simulink model "Model_2017_04_18"  (R2016a)
settings: Solver=VariableStepAuto  StartTime=0.0  StopTime=2  RelTol=1e-3
InitFcn:
  | parametriAM
values from neighbouring files (symbols this model uses):
  Imrn = 7.4    [parametriAM.m]
  Ismax = In*sqrt(2)    [parametriAM.m]
  J = 0.019    [parametriAM.m]    (also in podatki.m = 0.01)
  Ki_Imr = 1000    [parametriAM.m]
  Ki_tok = 5.0    (= 5)    [parametriAM.m]
  Kp_Imr = 100    [parametriAM.m]
  Kp_tok = 0.05    [parametriAM.m]
  Kp_wr = 50    [parametriAM.m]
  Lm = 0.0493    [parametriAM.m]    (also in podatki.m = 0.2342)
  Lr = 0.05315    [parametriAM.m]    (also in podatki.m = 0.2449)
  Ls = 0.05315    [parametriAM.m]    (also in podatki.m = 0.2449)
  Lst = sigma*Ls    (= 0.00742111947319)    [parametriAM.m]
  pp = 3    [parametriAM.m]    (also in podatki.m = 2)
  Rs = 0.594    [parametriAM.m]    (also in podatki.m = 3.7)
  sigma = 1 - 1/((1+sigmaR)*(1+sigmaS))    (= 0.13962595434)    [parametriAM.m]
  Tr = Lr/Rr    (= 0.0771407837446)    [parametriAM.m]
  Udc = Un*sqrt(2/3*2)    [parametriAM.m]
  wb_upper_limit_field_weaking = sqrt((Ls^2+Lst^2)/(2*Lst^2*Ls^2))*Un/Ismax    [parametriAM.m]
  wn = Udc/sqrt(Ls^2*(Imrn)^2+Lst^2*(Ismax^2-(Imrn)^2))    [maximalnaelipsa.m]    (also in parametriAM.m = Udc/sqrt(Ls^2*(Imrn)^2+Lst^2*(Ismax^2-(Imrn)^2))/pp/sqrt(2))
libraries: simulink x6
settings Model: Creator=Mitja1  LastModifiedBy=Mitja1

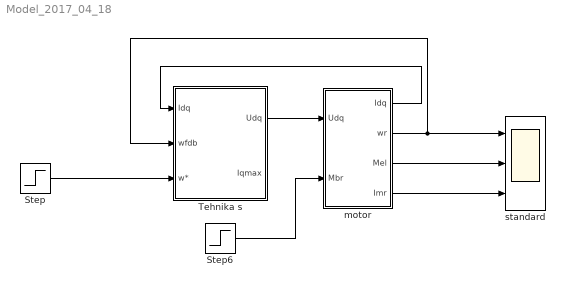
== system Model_2017_04_18 ==
  Step : Step  Time=0.05  After=4000/60*2*pi  SampleTime=0
  Step6 : Step  Time=0.5  After=2  SampleTime=0
  Tehnika s : Subsystem
  motor : Subsystem
  standard : Scope  NumInputPorts=3
  wires:
  motor/1(Idq) -> Tehnika s/1(Idq)
  motor/2(wr) -> Tehnika s/2(wfdb), standard/1
  motor/4(Imr) -> standard/3
  Tehnika s/1(Udq) -> motor/1(Udq)
  motor/3(Mel) -> standard/2
  Step6/1 -> motor/2(Mbr)
  Step/1 -> Tehnika s/3(w*)

== system Model_2017_04_18/Tehnika s ==
  Idq : Inport
  wfdb : Inport  Port=2
  w* : Inport  Port=3
  Gain2 : Gain  Gain=Udc
  M9 : ToWorkspace  VariableName=I_mr_sref  SampleTime=-1
      settings: Decimation=3  Save2DSignal=2-D array (concatenate along first dimension)
  Magnetilnireg : Subsystem
  Manual Switch : ManualSwitch
  Regulacija navora : Subsystem
  Subsystem : Subsystem
  Tok regulator : Subsystem
  Udq : Outport
  Iqmax : Outport  Port=2
  wires:
  Regulacija navora/1(iq*) -> Tok regulator/3(Iq)
  Regulacija navora/2(Iqmax) -> Iqmax/1
  Idq/1 -> Tok regulator/1(Idqdej), Regulacija navora/2(Idqdej), Subsystem/2(Idq), Magnetilnireg/1(Idqdej)
  w*/1 -> Subsystem/1(In1), Regulacija navora/1(w*)
  Tok regulator/1(Udq*) -> Gain2/1
  Gain2/1 -> Udq/1
  Magnetilnireg/1(Id*) -> Tok regulator/2(Id)
  Manual Switch/1 -> Magnetilnireg/2(Imr*)
  Subsystem/2(A) -> Manual Switch/1
  Subsystem/3(B) -> Manual Switch/2
  wfdb/1 -> Regulacija navora/3(wfdb)

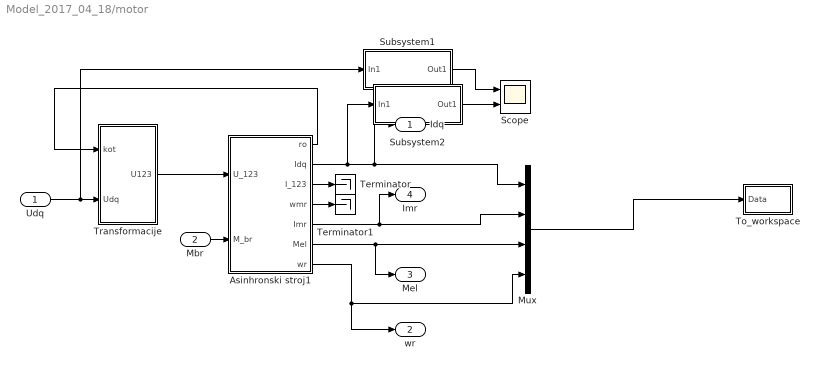
== system Model_2017_04_18/motor ==
  Udq : Inport
  Mbr : Inport  Port=2
  Asinhronski stroj1 : Subsystem  InitFcn=parametriAM
  Mux : Mux
  Scope : Scope  NumInputPorts=2
  Subsystem1 : Subsystem
  Subsystem2 : Subsystem
  Terminator : Terminator
  Terminator1 : Terminator
  To_workspace : Subsystem
  Transformacije : Subsystem
  Idq : Outport
  wr : Outport  Port=2
  Mel : Outport  Port=3
  Imr : Outport  Port=4
  wires:
  Mbr/1 -> Asinhronski stroj1/2(M_br)
  Asinhronski stroj1/6(Mel) -> Mux/3, Mel/1
  Asinhronski stroj1/7(wr) -> wr/1, Mux/4
  Asinhronski stroj1/5(Imr) -> Mux/2, Imr/1
  Udq/1 -> Subsystem1/1(In1), Transformacije/2(Udq)
  Transformacije/1(U123) -> Asinhronski stroj1/1(U_123)
  Asinhronski stroj1/1(ro) -> Transformacije/1(kot)
  Asinhronski stroj1/2(Idq) -> Subsystem2/1(In1), Idq/1, Mux/1
  Mux/1 -> To_workspace/1(Data)
  Asinhronski stroj1/4(wmr) -> Terminator1/1
  Asinhronski stroj1/3(I_123) -> Terminator/1
  Subsystem1/1(Out1) -> Scope/1
  Subsystem2/1(Out1) -> Scope/2

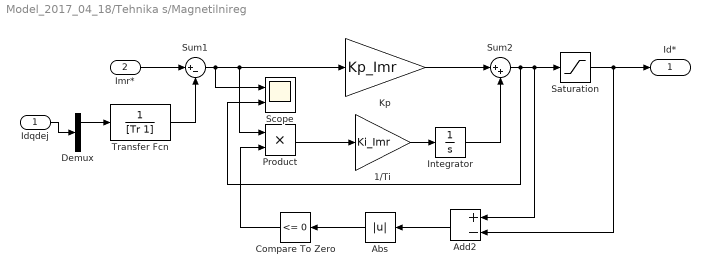
== system Model_2017_04_18/Tehnika s/Magnetilnireg ==
  Idqdej : Inport
  Imr* : Inport  Port=2
  1/Ti : Gain  Gain=Ki_Imr  SaturateOnIntegerOverflow=on  OutDataTypeStr=Inherit: Same as input  ParamDataTypeStr=Inherit: Same as input
  Abs : Abs  ZeroCross=off
  Add2 : Sum  Inputs=+-
  Compare To Zero : simulink/Logic and Bit Operations/Compare To Zero  relop=<=  OutDataTypeStr=boolean  ZeroCross=off
  Demux : Demux  Outputs=2
  Integrator : Integrator
  Kp : Gain  Gain=Kp_Imr  SaturateOnIntegerOverflow=on  OutDataTypeStr=Inherit: Same as input  ParamDataTypeStr=Inherit: Same as input
  Product : Product
  Saturation : Saturate  UpperLimit=Ismax  LowerLimit=-Ismax  ZeroCross=off
  Scope : Scope  NumInputPorts=2
  Sum1 : Sum  Inputs=|+-
  Sum2 : Sum  Inputs=|++
  Transfer Fcn : TransferFcn  Denominator=[Tr 1]
  Id* : Outport
  wires:
  Idqdej/1 -> Demux/1
  Transfer Fcn/1 -> Sum1/2
  Demux/1 -> Transfer Fcn/1
  Saturation/1 -> Id*/1, Add2/2
  Imr*/1 -> Sum1/1
  Integrator/1 -> Sum2/2
  Sum2/1 -> Saturation/1, Add2/1, Scope/2
  Compare To Zero/1 -> Product/2
  Kp/1 -> Sum2/1
  Product/1 -> 1/Ti/1
  1/Ti/1 -> Integrator/1
  Abs/1 -> Compare To Zero/1
  Add2/1 -> Abs/1
  Sum1/1 -> Kp/1, Product/1, Scope/1

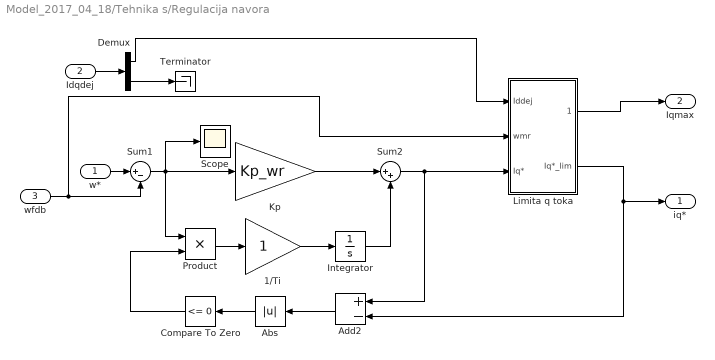
== system Model_2017_04_18/Tehnika s/Regulacija navora ==
  w* : Inport
  Idqdej : Inport  Port=2
  wfdb : Inport  Port=3
  1/Ti : Gain  SaturateOnIntegerOverflow=on  OutDataTypeStr=Inherit: Same as input  ParamDataTypeStr=Inherit: Same as input
  Abs : Abs
  Add2 : Sum  Inputs=+-
  Compare To Zero : simulink/Logic and Bit Operations/Compare To Zero  relop=<=  OutDataTypeStr=boolean
  Demux : Demux  Outputs=2
  Integrator : Integrator
  Kp : Gain  Gain=Kp_wr  SaturateOnIntegerOverflow=on  OutDataTypeStr=Inherit: Same as input  ParamDataTypeStr=Inherit: Same as input
  Limita q toka : Subsystem
  Product : Product
  Scope : Scope
  Sum1 : Sum  Inputs=|+-
  Sum2 : Sum  Inputs=|++
  Terminator : Terminator
  iq* : Outport
  Iqmax : Outport  Port=2
  wires:
  Demux/2 -> Terminator/1
  wfdb/1 -> Sum1/2, Limita q toka/2(wmr)
  Sum2/1 -> Add2/1, Limita q toka/3(Iq*)
  Demux/1 -> Limita q toka/1(Iddej)
  Limita q toka/1(Iqmaxlim) -> Iqmax/1
  Idqdej/1 -> Demux/1
  Limita q toka/2(Iq*_lim) -> Add2/2, iq*/1
  w*/1 -> Sum1/1
  Product/1 -> 1/Ti/1
  Compare To Zero/1 -> Product/2
  Kp/1 -> Sum2/1
  Abs/1 -> Compare To Zero/1
  Add2/1 -> Abs/1
  Integrator/1 -> Sum2/2
  Sum1/1 -> Scope/1, Kp/1, Product/1
  1/Ti/1 -> Integrator/1

== system Model_2017_04_18/Tehnika s/Subsystem ==
  In1 : Inport
  Idq : Inport  Port=2
  TechniqueA1 : Subsystem
  TechniqueA2 : Subsystem
  TechniqueB1 : Subsystem
  Nemec : Outport
  A : Outport  Port=2
  B : Outport  Port=3
  wires:
  In1/1 -> TechniqueA1/1(wmr), TechniqueB1/2(w), TechniqueA2/1(wmr)
  TechniqueA2/1(Nemec) -> Nemec/1
  Idq/1 -> TechniqueB1/1(Isdq)
  TechniqueB1/1(6.1-135) -> B/1
  TechniqueA1/1(6.1-126) -> A/1

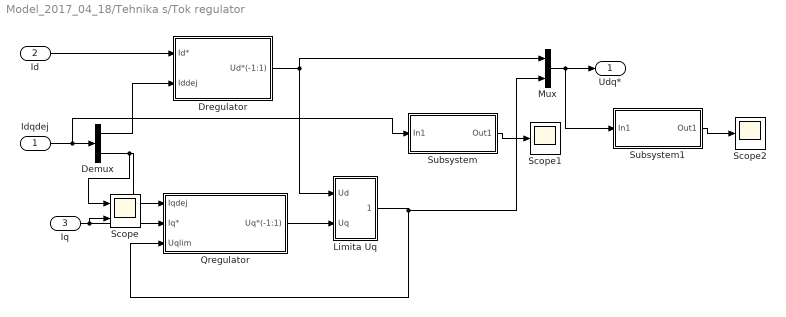
== system Model_2017_04_18/Tehnika s/Tok regulator ==
  Idqdej : Inport
  Id : Inport  Port=2
  Iq : Inport  Port=3
  Demux : Demux  Outputs=2
  Dregulator : Subsystem
  Limita Uq : Subsystem
  Mux : Mux  Inputs=2
  Qregulator : Subsystem
  Scope : Scope  NumInputPorts=2
  Scope1 : Scope
  Scope2 : Scope
  Subsystem : Subsystem
  Subsystem1 : Subsystem
  Udq* : Outport
  wires:
  Qregulator/1(Uq*(-1:1)) -> Limita Uq/2(Uq)
  Demux/2 -> Qregulator/1(Iqdej), Scope/1
  Iq/1 -> Qregulator/2(Iq*), Scope/2
  Demux/1 -> Dregulator/2(Iddej)
  Id/1 -> Dregulator/1(Id*)
  Dregulator/1(Ud*(-1:1)) -> Limita Uq/1(Ud), Mux/1
  Limita Uq/1(Uq_lim) -> Mux/2, Qregulator/3(Uqlim)
  Idqdej/1 -> Subsystem/1(In1), Demux/1
  Mux/1 -> Subsystem1/1(In1), Udq*/1
  Subsystem/1(Out1) -> Scope1/1
  Subsystem1/1(Out1) -> Scope2/1

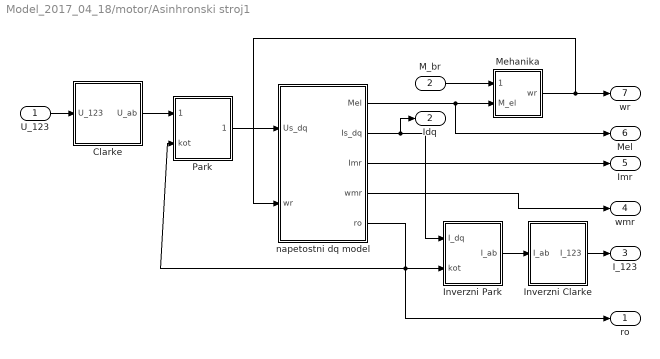
== system Model_2017_04_18/motor/Asinhronski stroj1 ==
  U_123 : Inport
  M_br : Inport  Port=2
  Clarke : Subsystem
  Inverzni Clarke : Subsystem
  Inverzni Park : Subsystem
  Mehanika : Subsystem
  Park : Subsystem
  napetostni dq model : Subsystem
  ro : Outport
  Idq : Outport  Port=2
  I_123 : Outport  Port=3
  wmr : Outport  Port=4
  Imr : Outport  Port=5
  Mel : Outport  Port=6
  wr : Outport  Port=7
  wires:
  Inverzni Park/1(I_ab) -> Inverzni Clarke/1(I_ab)
  Clarke/1(U_ab) -> Park/1(U_ab)
  Mehanika/1(wr) -> napetostni dq model/2(wr), wr/1
  M_br/1 -> Mehanika/1(M_br)
  napetostni dq model/1(Mel) -> Mel/1, Mehanika/2(M_el)
  Inverzni Clarke/1(I_123) -> I_123/1
  napetostni dq model/4(wmr) -> wmr/1
  napetostni dq model/3(Imr) -> Imr/1
  U_123/1 -> Clarke/1(U_123)
  napetostni dq model/2(Is_dq) -> Idq/1, Inverzni Park/1(I_dq)
  napetostni dq model/5(ro) -> ro/1, Park/2(kot), Inverzni Park/2(kot)
  Park/1(U_dq) -> napetostni dq model/1(Us_dq)

== system Model_2017_04_18/motor/Subsystem1 ==
  In1 : Inport
  Abs : Abs
  Demux1 : Demux  Outputs=2
  Real-Imag to Complex : RealImagToComplex
  Out1 : Outport
  wires:
  Demux1/1 -> Real-Imag to Complex/1
  Abs/1 -> Out1/1
  Demux1/2 -> Real-Imag to Complex/2
  Real-Imag to Complex/1 -> Abs/1
  In1/1 -> Demux1/1

== system Model_2017_04_18/motor/Subsystem2 ==
  In1 : Inport
  Abs : Abs
  Demux1 : Demux  Outputs=2
  Real-Imag to Complex : RealImagToComplex
  Out1 : Outport
  wires:
  In1/1 -> Demux1/1
  Real-Imag to Complex/1 -> Abs/1
  Demux1/2 -> Real-Imag to Complex/2
  Abs/1 -> Out1/1
  Demux1/1 -> Real-Imag to Complex/1

== system Model_2017_04_18/motor/To_workspace ==
  Data : Inport
  Demux : Demux
  M1 : ToWorkspace  VariableName=Idq_s  SampleTime=-1
      settings: Decimation=3  Save2DSignal=2-D array (concatenate along first dimension)
  M10 : ToWorkspace  VariableName=w_fdb_s  SampleTime=-1
      settings: Decimation=3  Save2DSignal=2-D array (concatenate along first dimension)
  M5 : ToWorkspace  VariableName=M_el_s  SampleTime=-1
      settings: Decimation=3  Save2DSignal=2-D array (concatenate along first dimension)
  M9 : ToWorkspace  VariableName=I_mr_s  SampleTime=-1
      settings: Decimation=3  Save2DSignal=2-D array (concatenate along first dimension)
  wires:
  Demux/4 -> M10/1
  Data/1 -> Demux/1
  Demux/1 -> M1/1
  Demux/2 -> M9/1
  Demux/3 -> M5/1

== system Model_2017_04_18/motor/Transformacije ==
  kot : Inport
  Udq : Inport  Port=2
  Inverzni Clarke : Subsystem
  Inverzni Park : Subsystem
  U123 : Outport
  wires:
  Inverzni Clarke/1(U_123) -> U123/1
  kot/1 -> Inverzni Park/1(kot)
  Inverzni Park/1(U_ab) -> Inverzni Clarke/1(U_ab)
  Udq/1 -> Inverzni Park/2(U_dq)

== system Model_2017_04_18/Tehnika s/Regulacija navora/Limita q toka ==
  Iddej : Inport
  wmr : Inport  Port=2
  Iq* : Inport  Port=3
  Gain : Gain  Gain=-1
  MinMax : MinMax  Inputs=2
  Saturation napetost : simulink/Discontinuities/Saturation Dynamic  OutMin=[]  OutMax=[]  OutDataTypeStr=Inherit: Same as second input  OutDataType=fixdt(1, 16)  OutScaling=2^-10  DoSatur=off
  Scope : Scope  NumInputPorts=2
  napetostna limita : Subsystem
  tokovna : Subsystem
  Iqmaxlim : Outport
  Iq*_lim : Outport  Port=2
  wires:
  tokovna/1(high) -> MinMax/2
  napetostna limita/1(high) -> MinMax/1
  Gain/1 -> Saturation napetost/3
  Saturation napetost/1 -> Iq*_lim/1
  Iq*/1 -> Saturation napetost/2
  MinMax/1 -> Gain/1, Iqmaxlim/1, Saturation napetost/1
  Iddej/1 -> tokovna/1(Id), napetostna limita/1(Iddej)
  wmr/1 -> napetostna limita/2(w)

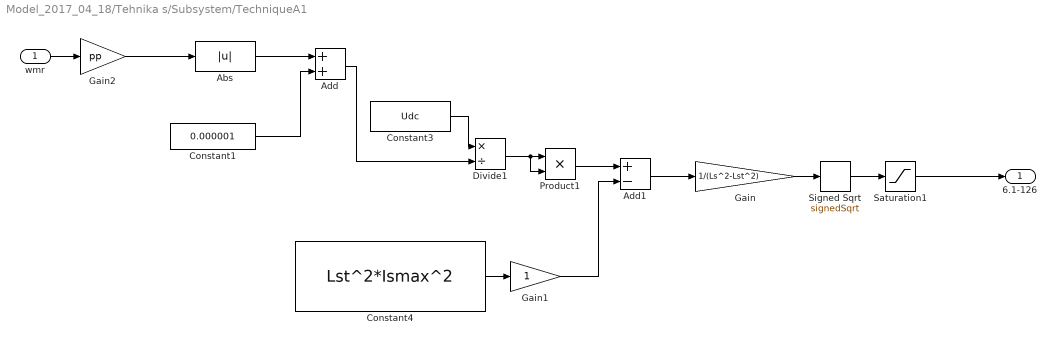
== system Model_2017_04_18/Tehnika s/Subsystem/TechniqueA1 ==
  wmr : Inport
  Abs : Abs
  Add : Sum
  Add1 : Sum  Inputs=+-
  Constant1 : Constant  Value=0.000001
  Constant3 : Constant  Value=Udc
  Constant4 : Constant  Value=Lst^2*Ismax^2
  Divide1 : Product  Inputs=*/
  Gain : Gain  Gain=1/(Ls^2-Lst^2)
  Gain1 : Gain
  Gain2 : Gain  Gain=pp
  Product1 : Product
  Saturation1 : Saturate  UpperLimit=+Imrn*sqrt(2)  LowerLimit=0
  Signed Sqrt : Sqrt  Operator=signedSqrt  OutputSignalType=real  SaturateOnIntegerOverflow=on
  6.1-126 : Outport
  wires:
  Add/1 -> Divide1/2
  Abs/1 -> Add/1
  Constant1/1 -> Add/2
  Constant3/1 -> Divide1/1
  Divide1/1 -> Product1/2, Product1/1
  Product1/1 -> Add1/1
  Saturation1/1 -> 6.1-126/1
  Add1/1 -> Gain/1
  Gain/1 -> Signed Sqrt/1
  Signed Sqrt/1 -> Saturation1/1
  Gain2/1 -> Abs/1
  Constant4/1 -> Gain1/1
  Gain1/1 -> Add1/2
  wmr/1 -> Gain2/1

== system Model_2017_04_18/Tehnika s/Subsystem/TechniqueA2 ==
  wmr : Inport
  Abs : Abs
  Add : Sum
  Constant : Constant  Value=wn
  Constant1 : Constant  Value=0.000001
  Constant2 : Constant  Value=Imrn*sqrt(2)
  Divide : Product  Inputs=*/
  Product : Product
  Saturation : Saturate  UpperLimit=+Imrn*sqrt(2)  LowerLimit=-Imrn*sqrt(2)
  Nemec : Outport
  wires:
  wmr/1 -> Abs/1
  Saturation/1 -> Nemec/1
  Constant1/1 -> Add/2
  Abs/1 -> Add/1
  Add/1 -> Divide/2
  Constant/1 -> Divide/1
  Product/1 -> Saturation/1
  Divide/1 -> Product/2
  Constant2/1 -> Product/1

== system Model_2017_04_18/Tehnika s/Subsystem/TechniqueB1 ==
  Isdq : Inport
  w : Inport  Port=2
  Add4 : Sum
  Const c : Subsystem
  Deljeno imenovalec 6.1-135 : Gain  Gain=1/(Ls^2-Lst^2)
  Demux : Demux  Outputs=2
  Gain4 : Gain  Gain=-Ls
  Gain6 : Gain  Gain=pp
  Korenski del : Subsystem
  Saturation : Saturate  UpperLimit=+Imrn*sqrt(2)  LowerLimit=-Imrn*sqrt(2)
  Scope : Scope
  Terminator : Terminator
  6.1-135 : Outport
  wires:
  Demux/1 -> Const c/1(Id)
  Demux/2 -> Terminator/1
  Saturation/1 -> 6.1-135/1
  Const c/1(c) -> Scope/1, Korenski del/1(c), Gain4/1
  Gain4/1 -> Add4/1
  Add4/1 -> Deljeno imenovalec 6.1-135/1
  Deljeno imenovalec 6.1-135/1 -> Saturation/1
  Isdq/1 -> Demux/1
  Korenski del/1(korenjen del) -> Add4/2
  w/1 -> Gain6/1
  Gain6/1 -> Korenski del/2(w)

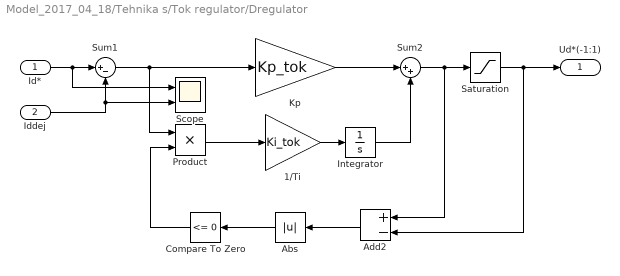
== system Model_2017_04_18/Tehnika s/Tok regulator/Dregulator ==
  Id* : Inport
  Iddej : Inport  Port=2
  1/Ti : Gain  Gain=Ki_tok  SaturateOnIntegerOverflow=on  OutDataTypeStr=Inherit: Same as input  ParamDataTypeStr=Inherit: Same as input
  Abs : Abs  ZeroCross=off
  Add2 : Sum  Inputs=+-
  Compare To Zero : simulink/Logic and Bit Operations/Compare To Zero  relop=<=  OutDataTypeStr=boolean  ZeroCross=off
  Integrator : Integrator
  Kp : Gain  Gain=Kp_tok  SaturateOnIntegerOverflow=on  OutDataTypeStr=Inherit: Same as input  ParamDataTypeStr=Inherit: Same as input
  Product : Product
  Saturation : Saturate  UpperLimit=0.990  LowerLimit=-0.99  ZeroCross=off
  Scope : Scope  NumInputPorts=2
  Sum1 : Sum  Inputs=|+-
  Sum2 : Sum  Inputs=|++
  Ud*(-1:1) : Outport
  wires:
  Saturation/1 -> Ud*(-1:1)/1, Add2/2
  Id*/1 -> Sum1/1, Scope/1
  Integrator/1 -> Sum2/2
  Sum2/1 -> Saturation/1, Add2/1
  Compare To Zero/1 -> Product/2
  Kp/1 -> Sum2/1
  Product/1 -> 1/Ti/1
  1/Ti/1 -> Integrator/1
  Iddej/1 -> Sum1/2, Scope/2
  Abs/1 -> Compare To Zero/1
  Add2/1 -> Abs/1
  Sum1/1 -> Kp/1, Product/1

== system Model_2017_04_18/Tehnika s/Tok regulator/Limita Uq ==
  Ud : Inport
  Uq : Inport  Port=2
  Abs : Abs
  Add : Sum  Inputs=+-
  Constant1 : Constant
  Gain : Gain  Gain=-1
  Product3 : Product
  Saturation Dynamic : simulink/Discontinuities/Saturation Dynamic  OutMin=[]  OutMax=[]  OutDataTypeStr=Inherit: Same as second input  OutDataType=fixdt(1, 16)  OutScaling=2^-10  DoSatur=on
  Scope : Scope
  Sqrt : Sqrt  SaturateOnIntegerOverflow=on
  Uq_lim : Outport
  wires:
  Abs/1 -> Gain/1, Saturation Dynamic/1, Scope/1
  Sqrt/1 -> Abs/1
  Add/1 -> Sqrt/1
  Product3/1 -> Add/2
  Gain/1 -> Saturation Dynamic/3
  Constant1/1 -> Add/1
  Saturation Dynamic/1 -> Uq_lim/1
  Uq/1 -> Saturation Dynamic/2
  Ud/1 -> Product3/2, Product3/1

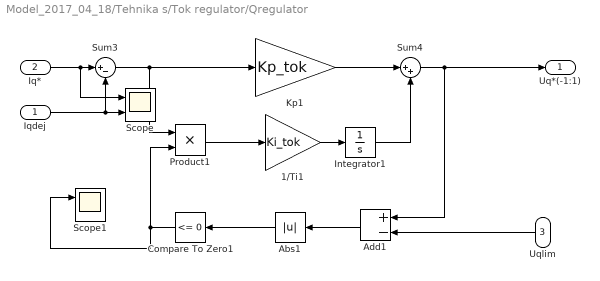
== system Model_2017_04_18/Tehnika s/Tok regulator/Qregulator ==
  Iqdej : Inport
  Iq* : Inport  Port=2
  Uqlim : Inport  Port=3
  1/Ti1 : Gain  Gain=Ki_tok  SaturateOnIntegerOverflow=on  OutDataTypeStr=Inherit: Same as input  ParamDataTypeStr=Inherit: Same as input
  Abs1 : Abs
  Add1 : Sum  Inputs=+-
  Compare To Zero1 : simulink/Logic and Bit Operations/Compare To Zero  relop=<=  OutDataTypeStr=boolean
  Integrator1 : Integrator
  Kp1 : Gain  Gain=Kp_tok  SaturateOnIntegerOverflow=on  OutDataTypeStr=Inherit: Same as input  ParamDataTypeStr=Inherit: Same as input
  Product1 : Product
  Scope : Scope  NumInputPorts=2
  Scope1 : Scope  NumInputPorts=2
  Sum3 : Sum  Inputs=|+-
  Sum4 : Sum  Inputs=|++
  Uq*(-1:1) : Outport
  wires:
  Sum4/1 -> Add1/1, Uq*(-1:1)/1
  Uqlim/1 -> Add1/2
  Iqdej/1 -> Scope/2, Sum3/2
  Abs1/1 -> Compare To Zero1/1
  1/Ti1/1 -> Integrator1/1
  Product1/1 -> 1/Ti1/1
  Compare To Zero1/1 -> Product1/2, Scope1/1
  Add1/1 -> Abs1/1
  Sum3/1 -> Product1/1, Kp1/1
  Integrator1/1 -> Sum4/2
  Kp1/1 -> Sum4/1
  Iq*/1 -> Scope/1, Sum3/1

== system Model_2017_04_18/Tehnika s/Tok regulator/Subsystem ==
  In1 : Inport
  Abs : Abs
  Demux1 : Demux  Outputs=2
  Real-Imag to Complex : RealImagToComplex
  Out1 : Outport
  wires:
  In1/1 -> Demux1/1
  Real-Imag to Complex/1 -> Abs/1
  Demux1/2 -> Real-Imag to Complex/2
  Abs/1 -> Out1/1
  Demux1/1 -> Real-Imag to Complex/1

== system Model_2017_04_18/Tehnika s/Tok regulator/Subsystem1 ==
  In1 : Inport
  Abs : Abs
  Demux1 : Demux  Outputs=2
  Real-Imag to Complex : RealImagToComplex
  Out1 : Outport
  wires:
  Demux1/1 -> Real-Imag to Complex/1
  Abs/1 -> Out1/1
  Demux1/2 -> Real-Imag to Complex/2
  Real-Imag to Complex/1 -> Abs/1
  In1/1 -> Demux1/1

== system Model_2017_04_18/motor/Asinhronski stroj1/Clarke ==
  U_123 : Inport
  ABC_ab1 : Subsystem
  Demux : Demux  Outputs=3
  Mux : Mux  Inputs=2
  U_ab : Outport
  wires:
  Mux/1 -> U_ab/1
  ABC_ab1/2(beta) -> Mux/2
  ABC_ab1/1(alfa) -> Mux/1
  Demux/3 -> ABC_ab1/3(C)
  Demux/2 -> ABC_ab1/2(B)
  Demux/1 -> ABC_ab1/1(A)
  U_123/1 -> Demux/1

== system Model_2017_04_18/motor/Asinhronski stroj1/Inverzni Clarke ==
  I_ab : Inport
  Demux : Demux  Outputs=2
  Mux : Mux  Inputs=3
  ab_ABC : Subsystem
  I_123 : Outport
  wires:
  ab_ABC/3(C) -> Mux/3
  ab_ABC/2(B) -> Mux/2
  ab_ABC/1(A) -> Mux/1
  Demux/2 -> ab_ABC/2(beta)
  Demux/1 -> ab_ABC/1(alfa)
  I_ab/1 -> Demux/1
  Mux/1 -> I_123/1

== system Model_2017_04_18/motor/Asinhronski stroj1/Inverzni Park ==
  I_dq : Inport
  kot : Inport  Port=2
  Demux : Demux  Outputs=2
  Mux : Mux  Inputs=2
  "Sum1 " : Sum  Inputs=+-  SaturateOnIntegerOverflow=on  InputSameDT=on  OutDataTypeStr=Inherit: Same as first input
  Sum2 : Sum  SaturateOnIntegerOverflow=on  InputSameDT=on  OutDataTypeStr=Inherit: Same as first input
  cos : Fcn  Expr=cos(u)
  sin : Fcn  Expr=sin(u)
  x_d*cos : Product  SaturateOnIntegerOverflow=on  RndMeth=Zero  InputSameDT=on  OutDataTypeStr=Inherit: Same as first input
  x_d*sin : Product  SaturateOnIntegerOverflow=on  RndMeth=Zero  InputSameDT=on  OutDataTypeStr=Inherit: Same as first input
  x_q*cos : Product  SaturateOnIntegerOverflow=on  RndMeth=Zero  InputSameDT=on  OutDataTypeStr=Inherit: Same as first input
  "x_q*sin " : Product  SaturateOnIntegerOverflow=on  RndMeth=Zero  InputSameDT=on  OutDataTypeStr=Inherit: Same as first input
  I_ab : Outport
  wires:
  Mux/1 -> I_ab/1
  I_dq/1 -> Demux/1
  Demux/1 -> x_d*sin/1, x_d*cos/1
  Demux/2 -> "x_q*sin "/1, x_q*cos/1
  cos/1 -> x_q*cos/2, x_d*cos/2
  sin/1 -> "x_q*sin "/2, x_d*sin/2
  x_d*cos/1 -> "Sum1 "/1
  "x_q*sin "/1 -> "Sum1 "/2
  x_q*cos/1 -> Sum2/2
  x_d*sin/1 -> Sum2/1
  "Sum1 "/1 -> Mux/1
  Sum2/1 -> Mux/2
  kot/1 -> cos/1, sin/1

== system Model_2017_04_18/motor/Asinhronski stroj1/Mehanika ==
  M_br : Inport
  M_el : Inport  Port=2
  Sum : Sum  Inputs=+-
  eq 2.19 : Subsystem
  wr : Outport
  wires:
  M_br/1 -> Sum/2
  Sum/1 -> eq 2.19/1(M)
  M_el/1 -> Sum/1
  eq 2.19/1(wr) -> wr/1

== system Model_2017_04_18/motor/Asinhronski stroj1/Park ==
  U_ab : Inport
  kot : Inport  Port=2
  Demux : Demux  Outputs=2
  Mux : Mux  Inputs=2
  "Sum1 " : Sum  SaturateOnIntegerOverflow=on  InputSameDT=on  OutDataTypeStr=Inherit: Same as first input
  Sum2 : Sum  Inputs=-+  SaturateOnIntegerOverflow=on  InputSameDT=on  OutDataTypeStr=Inherit: Same as first input
  cos : Fcn  Expr=cos(u)
  sin : Fcn  Expr=sin(u)
  x_a*cos : Product  SaturateOnIntegerOverflow=on  RndMeth=Zero  InputSameDT=on  OutDataTypeStr=Inherit: Same as first input
  x_a*sin : Product  SaturateOnIntegerOverflow=on  RndMeth=Zero  InputSameDT=on  OutDataTypeStr=Inherit: Same as first input
  x_b*cos : Product  SaturateOnIntegerOverflow=on  RndMeth=Zero  InputSameDT=on  OutDataTypeStr=Inherit: Same as first input
  "x_b*sin " : Product  SaturateOnIntegerOverflow=on  RndMeth=Zero  InputSameDT=on  OutDataTypeStr=Inherit: Same as first input
  U_dq : Outport
  wires:
  Mux/1 -> U_dq/1
  U_ab/1 -> Demux/1
  Demux/1 -> x_a*sin/1, x_a*cos/1
  Demux/2 -> "x_b*sin "/1, x_b*cos/1
  cos/1 -> x_b*cos/2, x_a*cos/2
  sin/1 -> "x_b*sin "/2, x_a*sin/2
  x_a*cos/1 -> "Sum1 "/1
  "x_b*sin "/1 -> "Sum1 "/2
  x_b*cos/1 -> Sum2/2
  x_a*sin/1 -> Sum2/1
  "Sum1 "/1 -> Mux/1
  Sum2/1 -> Mux/2
  kot/1 -> cos/1, sin/1

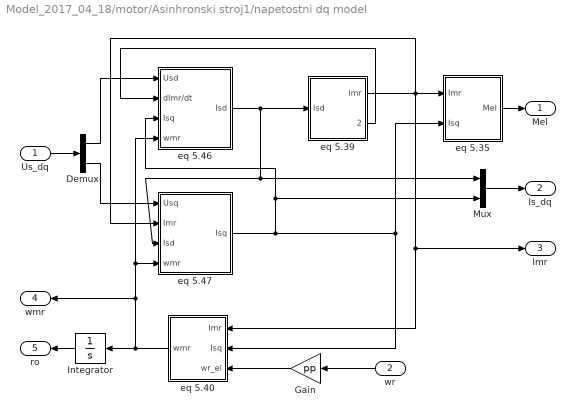
== system Model_2017_04_18/motor/Asinhronski stroj1/napetostni dq model ==
  Us_dq : Inport
  wr : Inport  Port=2
  Demux : Demux  Outputs=2
  Gain : Gain  Gain=pp
  Integrator : Integrator
  Mux : Mux  Inputs=2
  eq 5.35 : Subsystem
  eq 5.39 : Subsystem
  eq 5.40 : Subsystem
  eq 5.46 : Subsystem
  eq 5.47 : Subsystem
  Mel : Outport
  Is_dq : Outport  Port=2
  Imr : Outport  Port=3
  wmr : Outport  Port=4
  ro : Outport  Port=5
  wires:
  Gain/1 -> eq 5.40/3(wr_el)
  Mux/1 -> Is_dq/1
  Demux/2 -> eq 5.47/1(Usq)
  Demux/1 -> eq 5.46/1(Usd)
  Us_dq/1 -> Demux/1
  wr/1 -> Gain/1
  Integrator/1 -> ro/1
  eq 5.35/1(Mel) -> Mel/1
  eq 5.40/1(wmr) -> Integrator/1, wmr/1, eq 5.46/4(wmr), eq 5.47/4(wmr)
  eq 5.47/1(Isq) -> Mux/2, eq 5.46/3(Isq), eq 5.40/2(Isq), eq 5.35/2(Isq)
  eq 5.39/1(Imr) -> eq 5.47/2(Imr), Imr/1, eq 5.40/1(Imr), eq 5.35/1(Imr)
  eq 5.39/2(dImr/dt) -> eq 5.46/2(dImr/dt)
  eq 5.46/1(Isd) -> Mux/1, eq 5.47/3(Isd), eq 5.39/1(Isd)

== system Model_2017_04_18/motor/Transformacije/Inverzni Clarke ==
  U_ab : Inport
  Demux : Demux  Outputs=2
  Mux : Mux  Inputs=3
  ab_ABC : Subsystem
  U_123 : Outport
  wires:
  ab_ABC/3(C) -> Mux/3
  ab_ABC/2(B) -> Mux/2
  ab_ABC/1(A) -> Mux/1
  Demux/2 -> ab_ABC/2(beta)
  Demux/1 -> ab_ABC/1(alfa)
  U_ab/1 -> Demux/1
  Mux/1 -> U_123/1

== system Model_2017_04_18/motor/Transformacije/Inverzni Park ==
  kot : Inport
  U_dq : Inport  Port=2
  Demux : Demux  Outputs=2
  Mux : Mux  Inputs=2
  "Sum1 " : Sum  Inputs=+-  SaturateOnIntegerOverflow=on  InputSameDT=on  OutDataTypeStr=Inherit: Same as first input
  Sum2 : Sum  SaturateOnIntegerOverflow=on  InputSameDT=on  OutDataTypeStr=Inherit: Same as first input
  cos : Fcn  Expr=cos(u)
  sin : Fcn  Expr=sin(u)
  x_d*cos : Product  SaturateOnIntegerOverflow=on  RndMeth=Zero  InputSameDT=on  OutDataTypeStr=Inherit: Same as first input
  x_d*sin : Product  SaturateOnIntegerOverflow=on  RndMeth=Zero  InputSameDT=on  OutDataTypeStr=Inherit: Same as first input
  x_q*cos : Product  SaturateOnIntegerOverflow=on  RndMeth=Zero  InputSameDT=on  OutDataTypeStr=Inherit: Same as first input
  "x_q*sin " : Product  SaturateOnIntegerOverflow=on  RndMeth=Zero  InputSameDT=on  OutDataTypeStr=Inherit: Same as first input
  U_ab : Outport
  wires:
  Mux/1 -> U_ab/1
  U_dq/1 -> Demux/1
  Demux/1 -> x_d*sin/1, x_d*cos/1
  Demux/2 -> "x_q*sin "/1, x_q*cos/1
  cos/1 -> x_q*cos/2, x_d*cos/2
  sin/1 -> "x_q*sin "/2, x_d*sin/2
  x_d*cos/1 -> "Sum1 "/1
  "x_q*sin "/1 -> "Sum1 "/2
  x_q*cos/1 -> Sum2/2
  x_d*sin/1 -> Sum2/1
  "Sum1 "/1 -> Mux/1
  Sum2/1 -> Mux/2
  kot/1 -> cos/1, sin/1

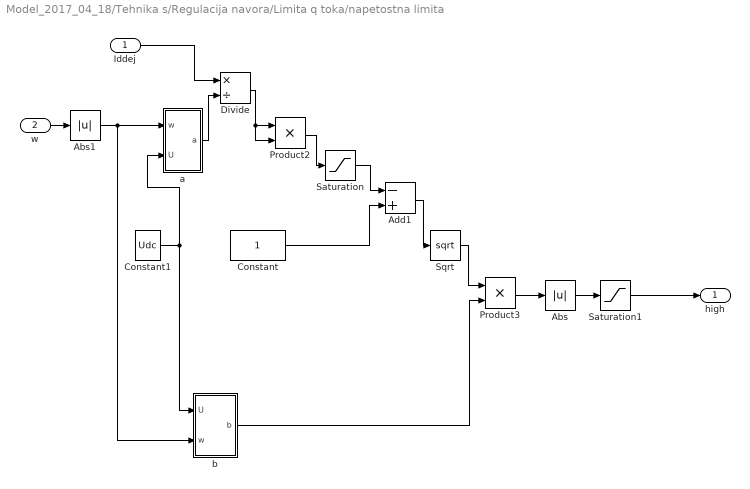
== system Model_2017_04_18/Tehnika s/Regulacija navora/Limita q toka/napetostna limita ==
  Iddej : Inport
  w : Inport  Port=2
  Abs : Abs
  Abs1 : Abs
  Add1 : Sum  Inputs=-+
  Constant : Constant
  Constant1 : Constant  Value=Udc
  Divide : Product  Inputs=*/
  Product2 : Product
  Product3 : Product
  Saturation : Saturate  UpperLimit=1  LowerLimit=0
  Saturation1 : Saturate  UpperLimit=Ismax  LowerLimit=0
  Sqrt : Sqrt  SaturateOnIntegerOverflow=on
  a : Subsystem
  b : Subsystem
  high : Outport
  wires:
  Constant1/1 -> a/2(U), b/1(U)
  Abs/1 -> Saturation1/1
  Saturation1/1 -> high/1
  Saturation/1 -> Add1/1
  Product2/1 -> Saturation/1
  Abs1/1 -> a/1(w), b/2(w)
  a/1(a) -> Divide/2
  b/1(b) -> Product3/2
  Add1/1 -> Sqrt/1
  Product3/1 -> Abs/1
  w/1 -> Abs1/1
  Constant/1 -> Add1/2
  Divide/1 -> Product2/2, Product2/1
  Iddej/1 -> Divide/1
  Sqrt/1 -> Product3/1

== system Model_2017_04_18/Tehnika s/Regulacija navora/Limita q toka/tokovna ==
  Id : Inport
  Abs : Abs
  Constant : Constant  Value=Ismax^2
  Product1 : Product
  Saturation : Saturate  UpperLimit=Ismax^2  LowerLimit=0
  Scope : Scope  NumInputPorts=2
  Sqrt : Sqrt  SaturateOnIntegerOverflow=on
  Subtract : Sum  Inputs=+-
  high : Outport
  wires:
  Saturation/1 -> Sqrt/1, Scope/2
  Subtract/1 -> Saturation/1, Scope/1
  Abs/1 -> high/1
  Product1/1 -> Subtract/2
  Constant/1 -> Subtract/1
  Id/1 -> Product1/1, Product1/2
  Sqrt/1 -> Abs/1

== system Model_2017_04_18/Tehnika s/Subsystem/TechniqueB1/Const c ==
  Id : Inport
  6.1-1 : TransferFcn  Numerator=[-Tr*Lm^2/Lr 0]  Denominator=[Tr 1]
  6.1-2 : TransferFcn  Denominator=[0.25 1]
  c : Outport
  wires:
  Id/1 -> 6.1-1/1
  6.1-1/1 -> 6.1-2/1
  6.1-2/1 -> c/1

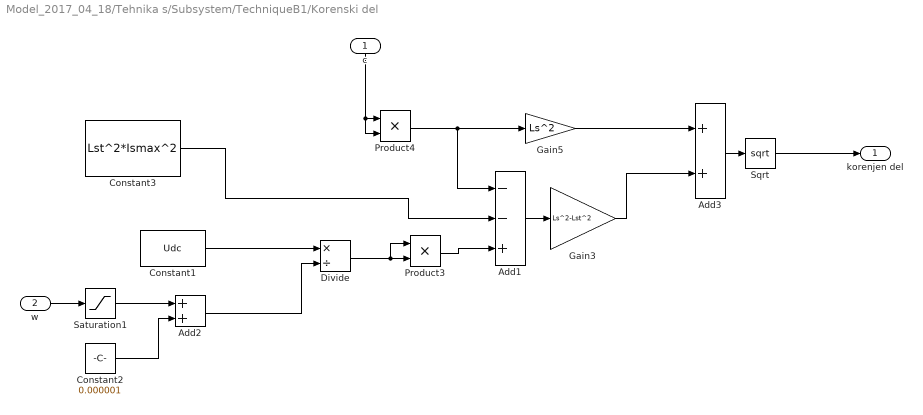
== system Model_2017_04_18/Tehnika s/Subsystem/TechniqueB1/Korenski del ==
  c : Inport
  w : Inport  Port=2
  Add1 : Sum  Inputs=--+
  Add2 : Sum
  Add3 : Sum
  Constant1 : Constant  Value=Udc
  Constant2 : Constant  Value=0.000001
  Constant3 : Constant  Value=Lst^2*Ismax^2
  Divide : Product  Inputs=*/
  Gain3 : Gain  Gain=Ls^2-Lst^2
  Gain5 : Gain  Gain=Ls^2
  Product3 : Product
  Product4 : Product
  Saturation1 : Saturate  UpperLimit=wb_upper_limit_field_weaking  LowerLimit=-wb_upper_limit_field_weaking
  Sqrt : Sqrt  SaturateOnIntegerOverflow=on
  korenjen del : Outport
  wires:
  c/1 -> Product4/2, Product4/1
  Product4/1 -> Add1/1, Gain5/1
  Saturation1/1 -> Add2/1
  Constant1/1 -> Divide/1
  Constant2/1 -> Add2/2
  Add1/1 -> Gain3/1
  Add2/1 -> Divide/2
  w/1 -> Saturation1/1
  Divide/1 -> Product3/1, Product3/2
  Product3/1 -> Add1/3
  Sqrt/1 -> korenjen del/1
  Add3/1 -> Sqrt/1
  Gain5/1 -> Add3/1
  Gain3/1 -> Add3/2
  Constant3/1 -> Add1/2

== system Model_2017_04_18/motor/Asinhronski stroj1/Clarke/ABC_ab1 ==
  A : Inport
  B : Inport  Port=2
  C : Inport  Port=3
  Gain1 : Gain  Gain=2
  Gain2 : Gain
  Gain24 : Gain  Gain=sqrt(3)/3
  Sum11 : Sum
  Terminator : Terminator
  alfa : Outport
  beta : Outport  Port=2
  wires:
  C/1 -> Terminator/1
  Gain1/1 -> Sum11/2
  B/1 -> Gain1/1
  Gain24/1 -> beta/1
  Gain2/1 -> alfa/1
  Sum11/1 -> Gain24/1
  A/1 -> Sum11/1, Gain2/1

== system Model_2017_04_18/motor/Asinhronski stroj1/Inverzni Clarke/ab_ABC ==
  alfa : Inport
  beta : Inport  Port=2
  Gain1 : Gain
  Gain2 : Gain  Gain=-0.5
  Gain25 : Gain  Gain=sqrt(3)/2
  Gain3 : Gain  Gain=sqrt(3)/2
  Gain4 : Gain  Gain=0.5
  Sum10 : Sum
  Sum11 : Sum  Inputs=--
  A : Outport
  B : Outport  Port=2
  C : Outport  Port=3
  wires:
  Gain3/1 -> Sum11/2
  beta/1 -> Gain25/1, Gain3/1
  Gain4/1 -> Sum11/1
  Gain25/1 -> Sum10/2
  Gain2/1 -> Sum10/1
  alfa/1 -> Gain1/1, Gain2/1, Gain4/1
  Gain1/1 -> A/1
  Sum10/1 -> B/1
  Sum11/1 -> C/1

== system Model_2017_04_18/motor/Asinhronski stroj1/Mehanika/eq 2.19 ==
  M : Inport
  Gain1 : Gain  Gain=1/J
  Integrator : Integrator
  wr : Outport
  wires:
  Integrator/1 -> wr/1
  M/1 -> Gain1/1
  Gain1/1 -> Integrator/1

== system Model_2017_04_18/motor/Asinhronski stroj1/napetostni dq model/eq 5.35 ==
  Imr : Inport
  Isq : Inport  Port=2
  Gain : Gain  Gain=3*pp/2
  Gain2 : Gain  Gain=Lm*Lm/Lr
  Product : Product  RndMeth=Zero
  Mel : Outport
  wires:
  Gain/1 -> Gain2/1
  Gain2/1 -> Mel/1
  Product/1 -> Gain/1
  Isq/1 -> Product/2
  Imr/1 -> Product/1

== system Model_2017_04_18/motor/Asinhronski stroj1/napetostni dq model/eq 5.39 ==
  Isd : Inport
  Gain : Gain  Gain=1/Tr
  Integrator : Integrator  InitialCondition=1e-3
  Sum : Sum  Inputs=|+-
  Imr : Outport
  dImr/dt : Outport  Port=2
  wires:
  Gain/1 -> dImr/dt/1, Integrator/1
  Sum/1 -> Gain/1
  Integrator/1 -> Sum/2, Imr/1
  Isd/1 -> Sum/1

== system Model_2017_04_18/motor/Asinhronski stroj1/napetostni dq model/eq 5.40 ==
  Imr : Inport
  Isq : Inport  Port=2
  wr_el : Inport  Port=3
  Divide : Product  Inputs=*/
  Gain2 : Gain  Gain=Tr
  Saturation : Saturate  UpperLimit=2*pi*50  LowerLimit=-2*pi*50
  Sum : Sum  Inputs=|++
  wmr : Outport
  wires:
  Saturation/1 -> Sum/1
  Sum/1 -> wmr/1
  wr_el/1 -> Sum/2
  Divide/1 -> Saturation/1  "ws"
  Gain2/1 -> Divide/2
  Imr/1 -> Gain2/1
  Isq/1 -> Divide/1

== system Model_2017_04_18/motor/Asinhronski stroj1/napetostni dq model/eq 5.46 ==
  Usd : Inport
  dImr/dt : Inport  Port=2
  Isq : Inport  Port=3
  wmr : Inport  Port=4
  Gain : Gain  Gain=1/(sigma*Ls)
  Gain1 : Gain  Gain=Rs
  Gain2 : Gain  Gain=(1-sigma)*Ls
  Gain3 : Gain  Gain=sigma*Ls
  Integrator : Integrator
  Product : Product  RndMeth=Zero
  Sum : Sum  Inputs=+--+
  Isd : Outport
  wires:
  Gain3/1 -> Sum/4
  Product/1 -> Gain3/1
  Isq/1 -> Product/1
  wmr/1 -> Product/2
  Gain2/1 -> Sum/3
  dImr/dt/1 -> Gain2/1
  Gain1/1 -> Sum/2
  Usd/1 -> Sum/1
  Sum/1 -> Gain/1
  Gain/1 -> Integrator/1
  Integrator/1 -> Gain1/1, Isd/1

== system Model_2017_04_18/motor/Asinhronski stroj1/napetostni dq model/eq 5.47 ==
  Usq : Inport
  Imr : Inport  Port=2
  Isd : Inport  Port=3
  wmr : Inport  Port=4
  Gain : Gain  Gain=1/(sigma*Ls)
  Gain1 : Gain  Gain=Rs
  Gain2 : Gain  Gain=(1-sigma)*Ls
  Gain3 : Gain  Gain=sigma*Ls
  Integrator : Integrator
  Product : Product  RndMeth=Zero
  Product1 : Product  RndMeth=Zero
  Sum : Sum  Inputs=+---
  Isq : Outport
  wires:
  Gain3/1 -> Sum/4
  Product1/1 -> Gain3/1
  Isd/1 -> Product1/2
  Gain2/1 -> Sum/3
  Product/1 -> Gain2/1
  wmr/1 -> Product1/1, Product/2
  Imr/1 -> Product/1
  Gain1/1 -> Sum/2
  Usq/1 -> Sum/1
  Sum/1 -> Gain/1
  Gain/1 -> Integrator/1
  Integrator/1 -> Gain1/1, Isq/1

== system Model_2017_04_18/motor/Transformacije/Inverzni Clarke/ab_ABC ==
  alfa : Inport
  beta : Inport  Port=2
  Gain1 : Gain
  Gain2 : Gain  Gain=-0.5
  Gain25 : Gain  Gain=sqrt(3)/2
  Gain3 : Gain  Gain=sqrt(3)/2
  Gain4 : Gain  Gain=0.5
  Sum10 : Sum
  Sum11 : Sum  Inputs=--
  A : Outport
  B : Outport  Port=2
  C : Outport  Port=3
  wires:
  Gain3/1 -> Sum11/2
  beta/1 -> Gain25/1, Gain3/1
  Gain4/1 -> Sum11/1
  Gain25/1 -> Sum10/2
  Gain2/1 -> Sum10/1
  alfa/1 -> Gain1/1, Gain2/1, Gain4/1
  Gain1/1 -> A/1
  Sum10/1 -> B/1
  Sum11/1 -> C/1

== system Model_2017_04_18/Tehnika s/Regulacija navora/Limita q toka/napetostna limita/a ==
  w : Inport
  U : Inport  Port=2
  Add3 : Sum
  Constant2 : Constant  Value=0.001
  Divide : Product  Inputs=*/
  Gain : Gain  Gain=1/Ls
  a : Outport
  wires:
  U/1 -> Gain/1
  Divide/1 -> a/1
  w/1 -> Add3/1
  Add3/1 -> Divide/2
  Constant2/1 -> Add3/2
  Gain/1 -> Divide/1

== system Model_2017_04_18/Tehnika s/Regulacija navora/Limita q toka/napetostna limita/b ==
  U : Inport
  w : Inport  Port=2
  Add4 : Sum
  Constant4 : Constant  Value=0.001
  Divide1 : Product  Inputs=*/
  Gain : Gain  Gain=1/Lst
  b : Outport
  wires:
  Gain/1 -> Divide1/1
  U/1 -> Gain/1
  Constant4/1 -> Add4/2
  Add4/1 -> Divide1/2
  w/1 -> Add4/1
  Divide1/1 -> b/1
